simulink model "mfordmodel_v1"  (R2023a)
settings: Solver=ode45  StartTime=0.0  StopTime=10.0  RelTol=1e-3  EnableMultiTasking=on
undefined symbols (not defined in the file): ABV_RATIO_SW, AC_OFF_DLY, ACLOD, AUTO_TRNS_SW, BRAKE_DNDT_X, BZZRPM, BZZRPM_ALT, BZZTM, BZZTM_ALT, CMD_LITOFF, CMD_STABLE, CO_ST_ECT__A, COOL_BASE, DAS_BKDLY_A, DAS_CNT, DAS_CTDLY, DAS_LC_SW__A, DASCLP_5INH, DASCTL, DASMHYST, DASMPH, DEBYCP, DES_BASE, DPNEU_MUL, DSDRPM_DN_TC, DSDRPM_OFF, DSDRPM_UP_TC, EDF_DELAY, EDFHP, ETC_CL_TP, ETC_HP, GR_CM_CREEP, HCAM_ACT_CLP, HEDFHP, HEDFRPM, HICAM_PS, IAC_CAL_SW, IAC_ER_TM1, IAC_ER_TM2, IAC_ER_TM4, IAC_HI_LIM__A, IAC_ISFL_OBD, IAC_KAM_SW, IAC_LO_LIM__A, IAC_MON_TM, IAC_OT_REQ, IAC_RUN_TM, IAC_TP_OBD, IAC_TR_DAS, IAC_TST_DC, ID_DAS__A, ID_NOVS__A, IDVS_CH__A, IDVS_SL__A, IPSI_SW, IPSIDLY, IS_DRBASE__A, IS_DRBASE_A__A, IS_NUBASE__A, IS_NUBASE_A__A ... (+35)
libraries: simulink x2
(part 5 of 12)

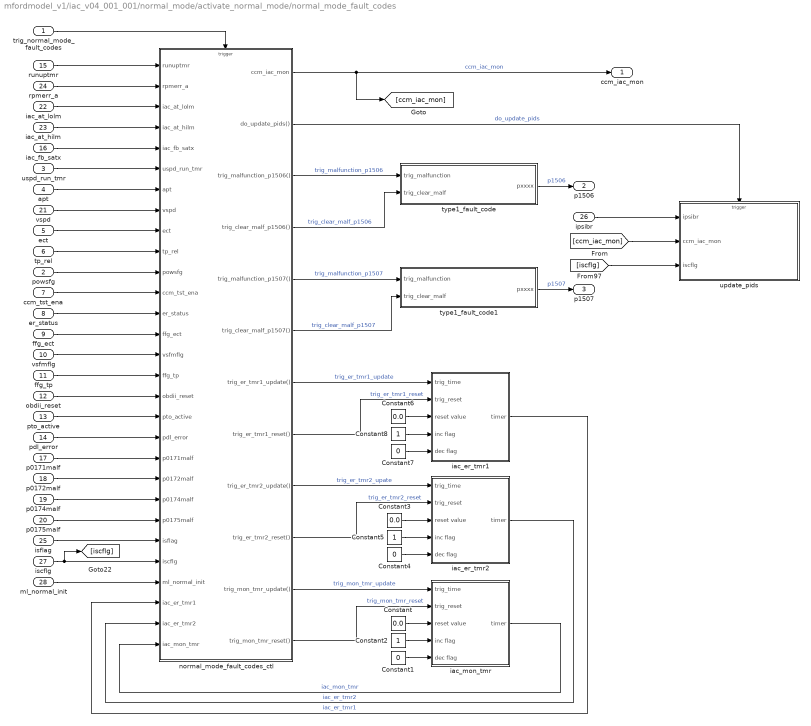
== system mfordmodel_v1/iac_v04_001_001/normal_mode/activate_normal_mode/normal_mode_fault_codes ==
  trig_normal_mode_fault_codes : Inport
  powsfg : Inport  Port=2
  uspd_run_tmr : Inport  Port=3
  apt : Inport  Port=4
  ect : Inport  Port=5
  tp_rel : Inport  Port=6
  ccm_tst_ena : Inport  Port=7
  er_status : Inport  Port=8
  ffg_ect : Inport  Port=9
  vsfmflg : Inport  Port=10
  ffg_tp : Inport  Port=11
  obdii_reset : Inport  Port=12
  pto_active : Inport  Port=13
  pdl_error : Inport  Port=14
  runuptmr : Inport  Port=15
  iac_fb_satx : Inport  Port=16
  p0171malf : Inport  Port=17
  p0172malf : Inport  Port=18
  p0174malf : Inport  Port=19
  p0175malf : Inport  Port=20
  vspd : Inport  Port=21
  iac_at_lolm : Inport  Port=22
  iac_at_hilm : Inport  Port=23
  rpmerr_a : Inport  Port=24
  isflag : Inport  Port=25
  ipsibr : Inport  Port=26
  iscflg : Inport  Port=27
  ml_normal_init : Inport  Port=28
  Constant : Constant  Value=0.0
  Constant1 : Constant  Value=0
  Constant2 : Constant
  Constant3 : Constant  Value=0.0
  Constant4 : Constant  Value=0
  Constant5 : Constant
  Constant6 : Constant  Value=0.0
  Constant7 : Constant  Value=0
  Constant8 : Constant
  iac_er_tmr1 : Subsystem  mask(TIMER){timer_name=iac_er_tmr1, init_value=0, clipped=off, tmin=, tmax=, unit_str=seconds}
      mask prompts: timer_name "Enter Timer Name"; init_value "initial TIMER value (in seconds)"; clipped "Clip timer?"; tmin "Minimum clip"; tmax "Maximum clip"; unit_str "Select timer units"
      mask help: Acts as a timer. Can count up, down, hold, or reset to zero. The required inputs are a timer function call, a reset function call, a reset value, an increment flag, and a decrement flag. Timer initial value, max and min clip values and timer name are selected below.
      mask init: same as mfordmodel_v1/iac_v04_001_001/normal_mode/activate_feedforward/ac_ppm_tmr
      mask Help:
      | <b><font size="+2">Input/Output Ports</font></b><br>
      | <p>
      | <b>Trig_timer:</b><br>
      | Connect a function call input to the 'trig_timer' port.  A function call passed through this port will activate the TIMER tool.  Activation updates the TIMER output.
      | <p>
      | <b>Trig_reset:</b><br>
      | Connect a function call input to the 'trig_reset' port.  A function call passed through this port will activate the TIMER tool.  Activation resets the TIMER output to the value passed to the 'reset_value' port.
      | <p>
      | <b>Reset_value:</b><br>
      | When 'trig_reset' is activated, the TIMER value will be reset to the real value passed to this input.
      | <p>
      | <b>Increment_flag and decrement_flag:</b><br>
      | If 'increment_flag' is 1 and 'decrement_flag' is 0, TIMER counts up.
      | If 'decrement_flag' is 1 and 'increment_flag' is 0, TIMER counts down.
      | If the flags are both 0 or both 1, TIMER holds its current value.
      | <p>
      | <b><font size="+2">Parameter Selection:</font></b>
      | <p>
      | <b>Initial TIMER Value:</b><br>
      | TIMER will begin at specified value.  Enter in seconds.
      mask TypeOptions unit_str: seconds | milliseconds
      mask Display:
      | plot( [0.3 0.45 0.55 0.7], [0.4 0.4 0.6 0.6])
      | plot( [ .475 .435 .415  .4 .4  .415 .435 .475  .525 .565 .585 .6 .6  ...
      | .585 .565 .525 .475], [.9  .885 .865  .825 .775 .735 .715  .7 .7 ...
      | .715 .735 .775 .825  .865 .885 .9 .9] )
      | plot( [.5 .5], [.89 .87])
      | plot( [.5 .5], [.71 .73])
      | plot( [.41 .43], [.8 .8])
      | plot( [.57 .59], [.8 .8])
      | plot( [.5 .5], [.8 .89])
      | plot( [.49 .5 .51], [.88 .89 .88] )
      | plot( [.5 .555], [.8 .825] )
      | plot( [.535 .555 .555], [.825 .825 .815])
      | text(0.35, 0.35, min_text)
      | text(0.6, 0.7,max_text)
      | text( 0.35, .95, timer_name)
  iac_er_tmr2 : Subsystem  mask(TIMER){timer_name=iac_er_tmr2, init_value=0, clipped=off, tmin=, tmax=, unit_str=seconds}
      mask prompts: timer_name "Enter Timer Name"; init_value "initial TIMER value (in seconds)"; clipped "Clip timer?"; tmin "Minimum clip"; tmax "Maximum clip"; unit_str "Select timer units"
      mask help: Acts as a timer. Can count up, down, hold, or reset to zero. The required inputs are a timer function call, a reset function call, a reset value, an increment flag, and a decrement flag. Timer initial value, max and min clip values and timer name are selected below.
      mask init: same as mfordmodel_v1/iac_v04_001_001/normal_mode/activate_feedforward/ac_ppm_tmr
      mask Help:
      | <b><font size="+2">Input/Output Ports</font></b><br>
      | <p>
      | <b>Trig_timer:</b><br>
      | Connect a function call input to the 'trig_timer' port.  A function call passed through this port will activate the TIMER tool.  Activation updates the TIMER output.
      | <p>
      | <b>Trig_reset:</b><br>
      | Connect a function call input to the 'trig_reset' port.  A function call passed through this port will activate the TIMER tool.  Activation resets the TIMER output to the value passed to the 'reset_value' port.
      | <p>
      | <b>Reset_value:</b><br>
      | When 'trig_reset' is activated, the TIMER value will be reset to the real value passed to this input.
      | <p>
      | <b>Increment_flag and decrement_flag:</b><br>
      | If 'increment_flag' is 1 and 'decrement_flag' is 0, TIMER counts up.
      | If 'decrement_flag' is 1 and 'increment_flag' is 0, TIMER counts down.
      | If the flags are both 0 or both 1, TIMER holds its current value.
      | <p>
      | <b><font size="+2">Parameter Selection:</font></b>
      | <p>
      | <b>Initial TIMER Value:</b><br>
      | TIMER will begin at specified value.  Enter in seconds.
      mask TypeOptions unit_str: seconds | milliseconds
      mask Display:
      | plot( [0.3 0.45 0.55 0.7], [0.4 0.4 0.6 0.6])
      | plot( [ .475 .435 .415  .4 .4  .415 .435 .475  .525 .565 .585 .6 .6  ...
      | .585 .565 .525 .475], [.9  .885 .865  .825 .775 .735 .715  .7 .7 ...
      | .715 .735 .775 .825  .865 .885 .9 .9] )
      | plot( [.5 .5], [.89 .87])
      | plot( [.5 .5], [.71 .73])
      | plot( [.41 .43], [.8 .8])
      | plot( [.57 .59], [.8 .8])
      | plot( [.5 .5], [.8 .89])
      | plot( [.49 .5 .51], [.88 .89 .88] )
      | plot( [.5 .555], [.8 .825] )
      | plot( [.535 .555 .555], [.825 .825 .815])
      | text(0.35, 0.35, min_text)
      | text(0.6, 0.7,max_text)
      | text( 0.35, .95, timer_name)
  iac_mon_tmr : Subsystem  mask(TIMER){timer_name=iac_mon_tmr, init_value=0, clipped=off, tmin=, tmax=, unit_str=seconds}
      mask prompts: timer_name "Enter Timer Name"; init_value "initial TIMER value (in seconds)"; clipped "Clip timer?"; tmin "Minimum clip"; tmax "Maximum clip"; unit_str "Select timer units"
      mask help: Acts as a timer. Can count up, down, hold, or reset to zero. The required inputs are a timer function call, a reset function call, a reset value, an increment flag, and a decrement flag. Timer initial value, max and min clip values and timer name are selected below.
      mask init: same as mfordmodel_v1/iac_v04_001_001/normal_mode/activate_feedforward/ac_ppm_tmr
      mask Help:
      | <b><font size="+2">Input/Output Ports</font></b><br>
      | <p>
      | <b>Trig_timer:</b><br>
      | Connect a function call input to the 'trig_timer' port.  A function call passed through this port will activate the TIMER tool.  Activation updates the TIMER output.
      | <p>
      | <b>Trig_reset:</b><br>
      | Connect a function call input to the 'trig_reset' port.  A function call passed through this port will activate the TIMER tool.  Activation resets the TIMER output to the value passed to the 'reset_value' port.
      | <p>
      | <b>Reset_value:</b><br>
      | When 'trig_reset' is activated, the TIMER value will be reset to the real value passed to this input.
      | <p>
      | <b>Increment_flag and decrement_flag:</b><br>
      | If 'increment_flag' is 1 and 'decrement_flag' is 0, TIMER counts up.
      | If 'decrement_flag' is 1 and 'increment_flag' is 0, TIMER counts down.
      | If the flags are both 0 or both 1, TIMER holds its current value.
      | <p>
      | <b><font size="+2">Parameter Selection:</font></b>
      | <p>
      | <b>Initial TIMER Value:</b><br>
      | TIMER will begin at specified value.  Enter in seconds.
      mask TypeOptions unit_str: seconds | milliseconds
      mask Display:
      | plot( [0.3 0.45 0.55 0.7], [0.4 0.4 0.6 0.6])
      | plot( [ .475 .435 .415  .4 .4  .415 .435 .475  .525 .565 .585 .6 .6  ...
      | .585 .565 .525 .475], [.9  .885 .865  .825 .775 .735 .715  .7 .7 ...
      | .715 .735 .775 .825  .865 .885 .9 .9] )
      | plot( [.5 .5], [.89 .87])
      | plot( [.5 .5], [.71 .73])
      | plot( [.41 .43], [.8 .8])
      | plot( [.57 .59], [.8 .8])
      | plot( [.5 .5], [.8 .89])
      | plot( [.49 .5 .51], [.88 .89 .88] )
      | plot( [.5 .555], [.8 .825] )
      | plot( [.535 .555 .555], [.825 .825 .815])
      | text(0.35, 0.35, min_text)
      | text(0.6, 0.7,max_text)
      | text( 0.35, .95, timer_name)
  normal_mode_fault_codes_ctl : Stateflow chart  TreatAsAtomicUnit=on
  type1_fault_code : Subsystem  mask(fault code){pcode=1506, ms=CCM}
      mask prompts: pcode "Code Number (e.g. 1234)"; ms "System ID"
      mask help: Gereric Fault Code - NOT functional
      mask init:
      | if (pcode == 'xxxx')
      | pcode_num = 0;
      | else
      | pcode_num = str2num(pcode);
      | end
      | mon_select=eval('ms');
      mask TypeOptions ms: CCM | CAT | PURG | SAIR | EGR | EGO | COOL | FCAP | P0456
      mask Display: fprintf('P%s\n%s',pcode,ms);
  type1_fault_code1 : Subsystem  mask(fault code){pcode=1507, ms=CCM}
      mask prompts: pcode "Code Number (e.g. 1234)"; ms "System ID"
      mask help: Gereric Fault Code - NOT functional
      mask init:
      | if (pcode == 'xxxx')
      | pcode_num = 0;
      | else
      | pcode_num = str2num(pcode);
      | end
      | mon_select=eval('ms');
      mask TypeOptions ms: CCM | CAT | PURG | SAIR | EGR | EGO | COOL | FCAP | P0456
      mask Display: fprintf('P%s\n%s',pcode,ms);
  update_pids : Subsystem  TreatAsAtomicUnit=on  mask(update_pids){}
      mask help: Update the specified PIDS.
      mask Display:
      | disp('
      | J2190_0x095D = ccm_iac_mon\n
      | J2190_0x097A = ipsibr               \n
      | J2190_0x097B = iscflg                \n')
  ccm_iac_mon : Outport
  p1506 : Outport  Port=2
  p1507 : Outport  Port=3
  wires:
  trig_normal_mode_fault_codes/1 -> normal_mode_fault_codes_ctl/Trigger
  normal_mode_fault_codes_ctl/7(trig_er_tmr1_update()) -> iac_er_tmr1/1(trig_time)  "trig_er_tmr1_update"
  normal_mode_fault_codes_ctl/8(trig_er_tmr1_reset()) -> iac_er_tmr1/2(trig_reset)  "trig_er_tmr1_reset"
  normal_mode_fault_codes_ctl/3(trig_malfunction_p1506()) -> type1_fault_code/1(trig_malfunction)  "trig_malfunction_p1506"
  normal_mode_fault_codes_ctl/4(trig_clear_malf_p1506()) -> type1_fault_code/2(trig_clear_malf)  "trig_clear_malf_p1506"
  normal_mode_fault_codes_ctl/5(trig_malfunction_p1507()) -> type1_fault_code1/1(trig_malfunction)  "trig_malfunction_p1507"
  normal_mode_fault_codes_ctl/6(trig_clear_malf_p1507()) -> type1_fault_code1/2(trig_clear_malf)  "trig_clear_malf_p1507"
  normal_mode_fault_codes_ctl/11(trig_mon_tmr_update()) -> iac_mon_tmr/1(trig_time)  "trig_mon_tmr_update"
  normal_mode_fault_codes_ctl/12(trig_mon_tmr_reset()) -> iac_mon_tmr/2(trig_reset)  "trig_mon_tmr_reset"
  normal_mode_fault_codes_ctl/10(trig_er_tmr2_reset()) -> iac_er_tmr2/2(trig_reset)  "trig_er_tmr2_reset"
  normal_mode_fault_codes_ctl/9(trig_er_tmr2_update()) -> iac_er_tmr2/1(trig_time)  "trig_er_tmr2_upate"
  iac_mon_tmr/1(timer) -> normal_mode_fault_codes_ctl/29(iac_mon_tmr)  "iac_mon_tmr"
  iac_er_tmr2/1(timer) -> normal_mode_fault_codes_ctl/28(iac_er_tmr2)  "iac_er_tmr2"
  iac_er_tmr1/1(timer) -> normal_mode_fault_codes_ctl/27(iac_er_tmr1)  "iac_er_tmr1"
  normal_mode_fault_codes_ctl/1(ccm_iac_mon) -> ccm_iac_mon/1, [ccm_iac_mon]  "ccm_iac_mon"
  Constant/1 -> iac_mon_tmr/3(reset value)
  Constant1/1 -> iac_mon_tmr/5(dec flag)
  Constant2/1 -> iac_mon_tmr/4(inc flag)
  Constant4/1 -> iac_er_tmr2/5(dec flag)
  Constant3/1 -> iac_er_tmr2/3(reset value)
  Constant5/1 -> iac_er_tmr2/4(inc flag)
  Constant6/1 -> iac_er_tmr1/3(reset value)
  Constant7/1 -> iac_er_tmr1/5(dec flag)
  Constant8/1 -> iac_er_tmr1/4(inc flag)
  normal_mode_fault_codes_ctl/2(do_update_pids()) -> update_pids/Trigger  "do_update_pids"
  iscflg/1 -> [iscflg], normal_mode_fault_codes_ctl/25(iscflg)
  ml_normal_init/1 -> normal_mode_fault_codes_ctl/26(ml_normal_init)
  runuptmr/1 -> normal_mode_fault_codes_ctl/1(runuptmr)
  rpmerr_a/1 -> normal_mode_fault_codes_ctl/2(rpmerr_a)
  iac_fb_satx/1 -> normal_mode_fault_codes_ctl/5(iac_fb_satx)
  iac_at_lolm/1 -> normal_mode_fault_codes_ctl/3(iac_at_lolm)
  iac_at_hilm/1 -> normal_mode_fault_codes_ctl/4(iac_at_hilm)
  isflag/1 -> normal_mode_fault_codes_ctl/24(isflag)
  powsfg/1 -> normal_mode_fault_codes_ctl/11(powsfg)
  uspd_run_tmr/1 -> normal_mode_fault_codes_ctl/6(uspd_run_tmr)
  apt/1 -> normal_mode_fault_codes_ctl/7(apt)
  vspd/1 -> normal_mode_fault_codes_ctl/8(vspd)
  ect/1 -> normal_mode_fault_codes_ctl/9(ect)
  tp_rel/1 -> normal_mode_fault_codes_ctl/10(tp_rel)
  ccm_tst_ena/1 -> normal_mode_fault_codes_ctl/12(ccm_tst_ena)
  er_status/1 -> normal_mode_fault_codes_ctl/13(er_status)
  ffg_ect/1 -> normal_mode_fault_codes_ctl/14(ffg_ect)
  vsfmflg/1 -> normal_mode_fault_codes_ctl/15(vsfmflg)
  ffg_tp/1 -> normal_mode_fault_codes_ctl/16(ffg_tp)
  obdii_reset/1 -> normal_mode_fault_codes_ctl/17(obdii_reset)
  pto_active/1 -> normal_mode_fault_codes_ctl/18(pto_active)
  pdl_error/1 -> normal_mode_fault_codes_ctl/19(pdl_error)
  p0171malf/1 -> normal_mode_fault_codes_ctl/20(p0171malf)
  p0172malf/1 -> normal_mode_fault_codes_ctl/21(p0172malf)
  p0174malf/1 -> normal_mode_fault_codes_ctl/22(p0174malf)
  p0175malf/1 -> normal_mode_fault_codes_ctl/23(p0175malf)
  type1_fault_code/1(pxxxx) -> p1506/1  "p1506"
  type1_fault_code1/1(pxxxx) -> p1507/1  "p1507"
  [iscflg] -> update_pids/3(iscflg)
  ipsibr/1 -> update_pids/1(ipsibr)
  [ccm_iac_mon] -> update_pids/2(ccm_iac_mon)

== system mfordmodel_v1/iac_v04_001_001/normal_mode/activate_normal_mode/output_flow_calc ==
  note: Note: Enable 'C-Like' bit
      | operations when Unit testing.
  note: UNIT TESTING NOTE: This module calculates "abv_flowrate"
      | and expects to see the modified value in the decision logic
      | "output_flow_calc_ctl" for determining the correct level of
      |  "iac_at_lolm & iac_at_hilm". Since "abv_flowrate" is a
      | merged parameter the model correctly has the merged
      | value "abv_flowrate_in" connected as an input to the decision
      | logic. However, since MatLab does not allow an input of a
      | merge block to be connected to more than one element,
      | it must  be manually wired to the state chart input for portions
      |  of the model unit test that utilize the limit logic.
      | ie, (P1506 & P1507 control).
  trig_output_flow_calc : Inport
  abv_percent : Inport  Port=2
  tr_res : Inport  Port=3
  tr_abs : Inport  Port=4
  pg_air : Inport  Port=5
  load : Inport  Port=6
  bp : Inport  Port=7
  engine_speed : Inport  Port=8
  act : Inport  Port=9
  map : Inport  Port=10
  abv_status : Inport  Port=11
  desmaf_pre : Inport  Port=12
  idle_ppm : Inport  Port=13
  isckam : Inport  Port=14
  ipsibr : Inport  Port=15
  isflag : Inport  Port=16
  abv_flowrate_in : Inport  Port=17
  abv_ratio_in : Inport  Port=18
  iac_inf_amb : Inport  Port=19
  desmaf_calc : Subsystem  TreatAsAtomicUnit=on
  output_flow_calc_ctl : Stateflow chart  TreatAsAtomicUnit=on
  tr_dsdrpm_calc : Subsystem  Description=test  TreatAsAtomicUnit=on  mask(tr_dsdrpm_calc){}
      mask help: TBD
      mask Display:
      | fprintf('ml_tr_dsdrpm_calc =
      | tr_abs - tr_res')
  abv_ratio : Outport
  abv_flowrate : Outport  Port=2
  iac_at_lolm : Outport  Port=3
  iac_at_hilm : Outport  Port=4
  iac_op_frac : Outport  Port=5
  wires:
  trig_output_flow_calc/1 -> output_flow_calc_ctl/Trigger
  output_flow_calc_ctl/2(iac_at_hilm) -> iac_at_hilm/1  "iac_at_hilm"
  output_flow_calc_ctl/1(iac_at_lolm) -> iac_at_lolm/1  "iac_at_lolm"
  abv_status/1 -> output_flow_calc_ctl/1(abv_status)
  output_flow_calc_ctl/9(do_tr_dsdrpm_calc()) -> tr_dsdrpm_calc/Trigger  "do_tr_dsdrpm_calc"
  tr_res/1 -> tr_dsdrpm_calc/2(tr_res)
  tr_abs/1 -> tr_dsdrpm_calc/1(tr_abs)
  tr_dsdrpm_calc/1(ml_tr_dsdrpm_calc) -> output_flow_calc_ctl/4(ml_tr_dsdrpm_calc), desmaf_calc/6(ml_tr_dsdrpm_calc)
  [do_desmaf_calc] -> desmaf_calc/Trigger
  output_flow_calc_ctl/3(ml_tr_dsdrpm_sw) -> desmaf_calc/1(ml_tr_dsdrpm_sw)  "ml_tr_dsdrpm_sw"
  output_flow_calc_ctl/5(ml_tr_das_sw) -> desmaf_calc/3(ml_tr_das_sw)  "ml_tr_das_sw"
  output_flow_calc_ctl/6(ml_ratio_sw) -> desmaf_calc/4(ml_ratio_sw)  "ml_ratio_sw"
  output_flow_calc_ctl/4(ml_flowrate_sw) -> desmaf_calc/2(ml_flowrate_sw)  "ml_flowrate_sw"
  output_flow_calc_ctl/8(do_desmaf_calc()) -> [do_desmaf_calc]  "do_desmaf_calc"
  isflag/1 -> output_flow_calc_ctl/2(isflag)
  output_flow_calc_ctl/7(ml_isflag_sw) -> desmaf_calc/5(ml_isflag_sw)  "ml_isflag_sw"
  abv_flowrate_in/1 -> output_flow_calc_ctl/3(abv_flowrate)
  desmaf_pre/1 -> desmaf_calc/7(desmaf_pre)
  ipsibr/1 -> desmaf_calc/9(ipsibr)
  idle_ppm/1 -> desmaf_calc/8(idle_ppm)
  isckam/1 -> desmaf_calc/10(isckam)
  map/1 -> desmaf_calc/11(map)
  bp/1 -> desmaf_calc/12(bp)
  engine_speed/1 -> desmaf_calc/15(engine_speed)
  load/1 -> desmaf_calc/16(load)
  act/1 -> desmaf_calc/14(act)
  pg_air/1 -> desmaf_calc/13(pg_air)
  abv_percent/1 -> desmaf_calc/17(abv_percent)
  abv_ratio_in/1 -> desmaf_calc/18(abv_ratio_in)
  desmaf_calc/1(iac_op_frac) -> iac_op_frac/1
  desmaf_calc/2(abv_ratio) -> abv_ratio/1
  desmaf_calc/3(abv_flowrate) -> abv_flowrate/1
  iac_inf_amb/1 -> desmaf_calc/19(iac_inf_amb)

== system mfordmodel_v1/iac_v04_001_001/normal_mode/iscflg_module/das_min_clip ==
  trig_das_min_clip_daspot : Inport
  trig_das_min_clip_prepos : Inport  Port=2
  dndsup : Inport  Port=3
  ndsflg : Inport  Port=4
  flg_crv_lk : Inport  Port=5
  dsdrpm : Inport  Port=6
  engine_speed : Inport  Port=7
  ptctfg : Inport  Port=8
  tfmflg : Inport  Port=9
  apt : Inport  Port=10
  flg_dasmnq : Inport  Port=11
  gear5tmr : Inport  Port=12
  das_ctr : Inport  Port=13
  dndt_das : Inport  Port=14
  iac_dlt_time : Inport  Port=15
  idle_ppm_in : Inport  Port=16
  gear5th : Inport  Port=17
  Gain : Gain  SaturateOnIntegerOverflow=on  OutDataTypeStr=Inherit: Same as input  ParamDataTypeStr=Inherit: Same as input
  Gain1 : Gain  SaturateOnIntegerOverflow=on  OutDataTypeStr=Inherit: Same as input  ParamDataTypeStr=Inherit: Same as input
  MinMax : MinMax  Function=max  Inputs=2  InputSameDT=on  SaturateOnIntegerOverflow=on
  Mux : Mux  Inputs=2
  das_min_clip_ctl : Stateflow chart  TreatAsAtomicUnit=on
  functions : Subsystem  TreatAsAtomicUnit=on
  daspot : Outport
  das_min_clp : Outport  Port=2
  idle_ppm : Outport  Port=3
  n_ratch : Outport  Port=4
  wires:
  das_min_clip_ctl/3(n_ratch) -> n_ratch/1, functions/1(n_ratch)  "n_ratch"
  MinMax/1 -> Gain1/1, Gain/1  "idle_ppm"
  Gain1/1 -> idle_ppm/1  "idle_ppm"
  Gain/1 -> daspot/1  "daspot"
  [idle_ppm_in] -> MinMax/2
  das_min_clip_ctl/1(das_min_clp) -> das_min_clp/1, MinMax/1  "das_min_clp"
  gear5th/1 -> das_min_clip_ctl/13(gear5th)
  idle_ppm_in/1 -> [idle_ppm_in], das_min_clip_ctl/12(idle_ppm_in)
  flg_crv_lk/1 -> das_min_clip_ctl/7(flg_crv_lk)
  tfmflg/1 -> das_min_clip_ctl/5(tfmflg)
  ptctfg/1 -> das_min_clip_ctl/3(ptctfg)
  dndsup/1 -> das_min_clip_ctl/1(dndsup)
  dndt_das/1 -> das_min_clip_ctl/11(dndt_das)
  das_ctr/1 -> das_min_clip_ctl/10(das_ctr)
  gear5tmr/1 -> das_min_clip_ctl/9(gear5tmr)
  flg_dasmnq/1 -> das_min_clip_ctl/8(flg_dasmnq)
  apt/1 -> das_min_clip_ctl/6(apt)
  ndsflg/1 -> das_min_clip_ctl/4(ndsflg)
  engine_speed/1 -> das_min_clip_ctl/2(engine_speed)
  iac_dlt_time/1 -> functions/3(iac_dlt_time)
  das_min_clip_ctl/2(dasl_min_clp) -> functions/2(dasl_min_clp)  "dasl_min_clp"
  functions/2(ml_rolav_llc) -> das_min_clip_ctl/21(ml_rolav_llc)
  functions/3(ml_rolav_l) -> das_min_clip_ctl/20(ml_rolav_l)
  functions/4(ml_rolav_h) -> das_min_clip_ctl/19(ml_rolav_h)
  functions/9(ml_fn894hlc) -> das_min_clip_ctl/14(ml_fn894hlc)
  functions/8(ml_fn894llc) -> das_min_clip_ctl/15(ml_fn894llc)
  functions/7(ml_fn894h) -> das_min_clip_ctl/16(ml_fn894h)
  functions/6(ml_fn894l) -> das_min_clip_ctl/17(ml_fn894l)
  functions/5(ml_fn894) -> das_min_clip_ctl/18(ml_fn894)
  dsdrpm/1 -> functions/4(dsdrpm)
  functions/1(ml_rolav_hlc) -> das_min_clip_ctl/22(ml_rolav_hlc)
  trig_das_min_clip_prepos/1 -> Mux/2
  trig_das_min_clip_daspot/1 -> Mux/1
  Mux/1 -> das_min_clip_ctl/Trigger
  das_min_clip_ctl/4(do_functions()) -> functions/Trigger  "do_functions"

== system mfordmodel_v1/iac_v04_001_001/normal_mode/iscflg_module/dashpot ==
  trig_activate_daspot_mode : Inport
  engine_speed : Inport  Port=2
  cttmr : Inport  Port=3
  apt : Inport  Port=4
  ndsflg : Inport  Port=5
  gr_cm : Inport  Port=6
  gr_old : Inport  Port=7
  pdl : Inport  Port=8
  vsbart : Inport  Port=9
  gr_cm_lst : Inport  Port=10
  igr_ds : Inport  Port=11
  flg_crv_lk : Inport  Port=12
  flg_sft_in : Inport  Port=13
  iac_dlt_time : Inport  Port=14
  idle_ppm_in : Inport  Port=15
  gear5th : Inport  Port=16
  dndt_das : Inport  Port=17
  ptctfg : Inport  Port=18
  Constant6 : Constant  Value=0
  Constant7 : Constant
  TIMER : Subsystem  mask(TIMER){timer_name=das_delay__A, init_value=0, clipped=on, tmin=0, tmax=inf, unit_str=seconds}
      mask prompts: timer_name "Enter Timer Name"; init_value "initial TIMER value (in seconds)"; clipped "Clip timer?"; tmin "Minimum clip"; tmax "Maximum clip"; unit_str "Select timer units"
      mask help: Acts as a timer. Can count up, down, hold, or reset to zero. The required inputs are a timer function call, a reset function call, a reset value, an increment flag, and a decrement flag. Timer initial value, max and min clip values and timer name are selected below.
      mask init: same as mfordmodel_v1/iac_v04_001_001/normal_mode/activate_feedforward/ac_ppm_tmr
      mask Help:
      | <b><font size="+2">Input/Output Ports</font></b><br>
      | <p>
      | <b>Trig_timer:</b><br>
      | Connect a function call input to the 'trig_timer' port.  A function call passed through this port will activate the TIMER tool.  Activation updates the TIMER output.
      | <p>
      | <b>Trig_reset:</b><br>
      | Connect a function call input to the 'trig_reset' port.  A function call passed through this port will activate the TIMER tool.  Activation resets the TIMER output to the value passed to the 'reset_value' port.
      | <p>
      | <b>Reset_value:</b><br>
      | When 'trig_reset' is activated, the TIMER value will be reset to the real value passed to this input.
      | <p>
      | <b>Increment_flag and decrement_flag:</b><br>
      | If 'increment_flag' is 1 and 'decrement_flag' is 0, TIMER counts up.
      | If 'decrement_flag' is 1 and 'increment_flag' is 0, TIMER counts down.
      | If the flags are both 0 or both 1, TIMER holds its current value.
      | <p>
      | <b><font size="+2">Parameter Selection:</font></b>
      | <p>
      | <b>Initial TIMER Value:</b><br>
      | TIMER will begin at specified value.  Enter in seconds.
      mask TypeOptions unit_str: seconds | milliseconds
      mask Display:
      | plot( [0.3 0.45 0.55 0.7], [0.4 0.4 0.6 0.6])
      | plot( [ .475 .435 .415  .4 .4  .415 .435 .475  .525 .565 .585 .6 .6  ...
      | .585 .565 .525 .475], [.9  .885 .865  .825 .775 .735 .715  .7 .7 ...
      | .715 .735 .775 .825  .865 .885 .9 .9] )
      | plot( [.5 .5], [.89 .87])
      | plot( [.5 .5], [.71 .73])
      | plot( [.41 .43], [.8 .8])
      | plot( [.57 .59], [.8 .8])
      | plot( [.5 .5], [.8 .89])
      | plot( [.49 .5 .51], [.88 .89 .88] )
      | plot( [.5 .555], [.8 .825] )
      | plot( [.535 .555 .555], [.825 .825 .815])
      | text(0.35, 0.35, min_text)
      | text(0.6, 0.7,max_text)
      | text( 0.35, .95, timer_name)
  activate_daspot_mode_ctl : Stateflow chart  TreatAsAtomicUnit=on
  daspot_calc : Subsystem  TreatAsAtomicUnit=on
  daspot_shift_trans_calc_ctl : Stateflow chart  TreatAsAtomicUnit=on
  function_calcs : Subsystem  TreatAsAtomicUnit=on
  trig_das_min_clip_daspot : Outport
  idle_ppm : Outport  Port=2
  das_ctr : Outport  Port=3
  wires:
  daspot_shift_trans_calc_ctl/2(das_tc__A) -> daspot_calc/5(das_tc__A)  "das_tc__A"
  daspot_shift_trans_calc_ctl/1(das_ppm__A) -> [das_ppm__A], daspot_calc/4(das_ppm__A)  "das_ppm__A"
  flg_crv_lk/1 -> activate_daspot_mode_ctl/8(flg_crv_lk)
  ptctfg/1 -> activate_daspot_mode_ctl/7(ptctfg)
  ndsflg/1 -> activate_daspot_mode_ctl/6(ndsflg)
  [engine_speed] -> activate_daspot_mode_ctl/9(engine_speed)
  [apt] -> activate_daspot_mode_ctl/10(apt)
  apt/1 -> [apt], daspot_shift_trans_calc_ctl/7(apt)
  [do_daspot_calc] -> daspot_calc/Trigger
  activate_daspot_mode_ctl/3(do_daspot_calc()) -> [do_daspot_calc]  "do_daspot_calc"
  [trig_dec_das_delay] -> TIMER/1(trig_time)
  activate_daspot_mode_ctl/5(trig_dec_das_delay()) -> [trig_dec_das_delay]  "trig_dec_das_delay"
  daspot_calc/1(idle_ppm) -> idle_ppm/1
  iac_dlt_time/1 -> daspot_calc/2(iac_dlt_time)
  idle_ppm_in/1 -> daspot_calc/3(idle_ppm_in)
  [trig_rst_das_delay] -> TIMER/2(trig_reset)
  Constant7/1 -> TIMER/5(dec flag)
  Constant6/1 -> TIMER/4(inc flag)
  daspot_shift_trans_calc_ctl/4(trig_rst_das_delay()) -> [trig_rst_das_delay]  "trig_rst_das_delay"
  [engine_speed] -> function_calcs/1(engine_speed)
  vsbart/1 -> [vsbart]
  engine_speed/1 -> [engine_speed]
  [vsbart] -> function_calcs/2(vsbart)
  daspot_shift_trans_calc_ctl/3(ml_das_delay) -> TIMER/3(reset value)  "ml_das_delay"
  TIMER/1(timer) -> [das_delay__A]  "das_delay__A"
  igr_ds/1 -> daspot_shift_trans_calc_ctl/1(igr_ds)
  pdl/1 -> daspot_shift_trans_calc_ctl/6(pdl)
  gr_cm/1 -> daspot_shift_trans_calc_ctl/4(gr_cm)
  flg_sft_in/1 -> daspot_shift_trans_calc_ctl/2(flg_sft_in)
  gr_cm_lst/1 -> daspot_shift_trans_calc_ctl/5(gr_cm_lst)
  gr_old/1 -> daspot_shift_trans_calc_ctl/3(gr_old)
  daspot_shift_trans_calc_ctl/5(do_function_calcs()) -> function_calcs/Trigger  "do_function_calcs"
  function_calcs/8(ml_fn899) -> daspot_shift_trans_calc_ctl/8(ml_fn899)
  function_calcs/7(ml_fnbo12) -> daspot_shift_trans_calc_ctl/9(ml_fnbo12)
  function_calcs/6(ml_fnbo13) -> daspot_shift_trans_calc_ctl/10(ml_fnbo13)
  function_calcs/5(ml_fnbo23) -> daspot_shift_trans_calc_ctl/11(ml_fnbo23)
  function_calcs/4(ml_fnbo24) -> daspot_shift_trans_calc_ctl/12(ml_fnbo24)
  function_calcs/3(ml_fnbo34) -> daspot_shift_trans_calc_ctl/13(ml_fnbo34)
  function_calcs/2(ml_fnbo35) -> daspot_shift_trans_calc_ctl/14(ml_fnbo35)
  function_calcs/1(ml_fnbo45) -> daspot_shift_trans_calc_ctl/15(ml_fnbo45)
  activate_daspot_mode_ctl/6(trig_daspot_shift_trans_calc()) -> daspot_shift_trans_calc_ctl/Trigger  "trig_daspot_shift_trans_calc"
  dndt_das/1 -> activate_daspot_mode_ctl/5(dndt_das)
  cttmr/1 -> activate_daspot_mode_ctl/4(cttmr)
  gear5th/1 -> activate_daspot_mode_ctl/3(gear5th)
  activate_daspot_mode_ctl/2(das_ctr) -> das_ctr/1  "das_ctr"
  activate_daspot_mode_ctl/4(trig_das_min_clip_daspot()) -> trig_das_min_clip_daspot/1  "trig_das_min_clip_daspot"
  activate_daspot_mode_ctl/1(ml_idle_ppm_sw) -> daspot_calc/1(ml_idle_ppm_sw)  "ml_idle_ppm_sw"
  trig_activate_daspot_mode/1 -> activate_daspot_mode_ctl/Trigger
  [das_delay__A] -> activate_daspot_mode_ctl/1(das_delay__A)
  [das_ppm__A] -> activate_daspot_mode_ctl/2(das_ppm__A)

== system mfordmodel_v1/iac_v04_001_001/normal_mode/iscflg_module/idle_drive_rpm_controller ==
  trig_idle_drive_rpm_controller : Inport
  ml_idrv_init_flg : Inport  Port=2
  iac_dlt_time : Inport  Port=3
  engine_speed : Inport  Port=4
  load : Inport  Port=5
  idle_drive_rpm_controller_ctl : Stateflow chart  TreatAsAtomicUnit=on
  idle_ppm_calc : Subsystem  TreatAsAtomicUnit=on
  idnerr_fil_calc : Subsystem  TreatAsAtomicUnit=on  mask(idnerr_fil_calc){}
      mask help: TBD
      mask Display:
      | disp('
      | ml_idnerr = (DSDRPM__A - engine_speed) \n\n
      | idnerr_fil = ROLAV (idnerr_fil, ml_idnerr,    \n
      | iac_dlt_time,  IDNERR_TC )       ')
  idle_ppm : Outport
  wires:
  idnerr_fil_calc/1(ml_idnerr) -> idle_ppm_calc/1(ml_idnerr)
  [do_idle_ppm_calc] -> idle_ppm_calc/Trigger
  idle_ppm_calc/1(idle_ppm) -> idle_ppm/1
  idle_ppm_calc/2(idnerr__A) -> [idnerr__A]
  [ml_init_sw] -> idle_ppm_calc/3(ml_init_sw)
  [ml_idnerr_sw] -> idle_ppm_calc/4(ml_idnerr_sw)
  load/1 -> idle_ppm_calc/5(load)
  idnerr_fil_calc/2(idnerr_fil) -> idle_drive_rpm_controller_ctl/2(idnerr_fil), idle_ppm_calc/2(idnerr_fil)
  iac_dlt_time/1 -> idnerr_fil_calc/3(iac_dlt_time)
  engine_speed/1 -> idnerr_fil_calc/2(engine_speed)
  [do_idnerr_fil_calc] -> idnerr_fil_calc/Trigger
  idle_drive_rpm_controller_ctl/1(ml_init_sw) -> idnerr_fil_calc/1(ml_init_sw), [ml_init_sw]  "ml_init_sw"
  idle_drive_rpm_controller_ctl/2(ml_idnerr_sw) -> [ml_idnerr_sw]  "ml_idnerr_sw"
  trig_idle_drive_rpm_controller/1 -> idle_drive_rpm_controller_ctl/Trigger
  ml_idrv_init_flg/1 -> idle_drive_rpm_controller_ctl/1(ml_idrv_init_flg)
  idle_drive_rpm_controller_ctl/3(do_idle_ppm_calc()) -> [do_idle_ppm_calc]  "do_idle_ppm_calc"
  idle_drive_rpm_controller_ctl/4(do_idnerr_fil_calc()) -> [do_idnerr_fil_calc]  "do_idnerr_fil_calc"
  [idnerr__A] -> idle_drive_rpm_controller_ctl/3(idnerr__A)

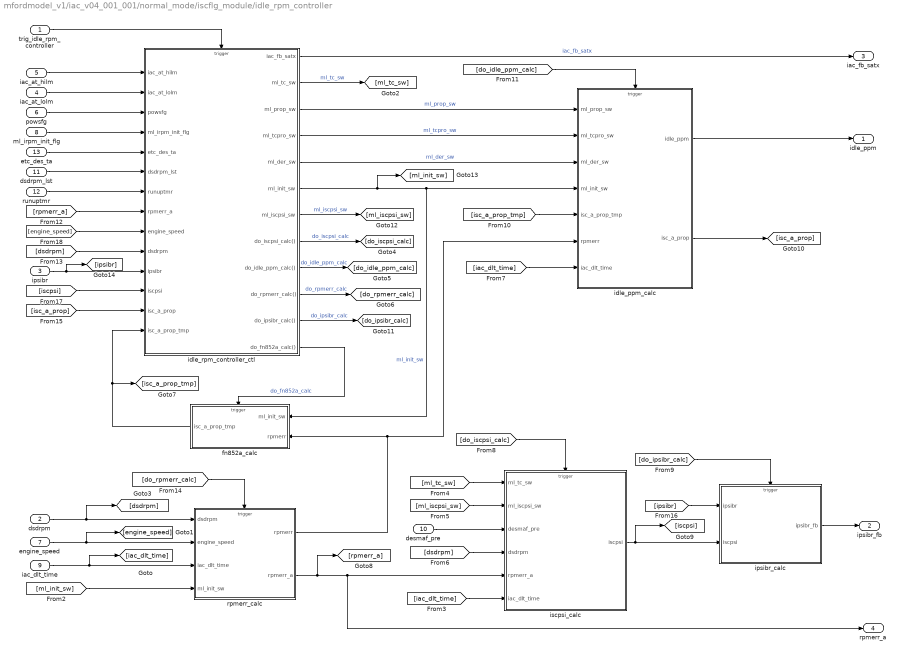
== system mfordmodel_v1/iac_v04_001_001/normal_mode/iscflg_module/idle_rpm_controller ==
  trig_idle_rpm_controller : Inport
  dsdrpm : Inport  Port=2
  ipsibr : Inport  Port=3
  iac_at_lolm : Inport  Port=4
  iac_at_hilm : Inport  Port=5
  powsfg : Inport  Port=6
  engine_speed : Inport  Port=7
  ml_irpm_init_flg : Inport  Port=8
  iac_dlt_time : Inport  Port=9
  desmaf_pre : Inport  Port=10
  dsdrpm_lst : Inport  Port=11
  runuptmr : Inport  Port=12
  etc_des_ta : Inport  Port=13
  fn852a_calc : Subsystem  TreatAsAtomicUnit=on
  idle_ppm_calc : Subsystem  TreatAsAtomicUnit=on
  idle_rpm_controller_ctl : Stateflow chart  TreatAsAtomicUnit=on
  ipsibr_calc : Subsystem  TreatAsAtomicUnit=on  mask(ipsibr_calc){}
      mask help: Calculate ipsibr feedback value.
      mask Display:
      | disp('
      | ipsibr_fb = ipsibr + iscpsi\n
      | ')
  iscpsi_calc : Subsystem  TreatAsAtomicUnit=on
  rpmerr_calc : Subsystem  TreatAsAtomicUnit=on
  idle_ppm : Outport
  ipsibr_fb : Outport  Port=2
  iac_fb_satx : Outport  Port=3
  rpmerr_a : Outport  Port=4
  wires:
  [engine_speed] -> idle_rpm_controller_ctl/9(engine_speed)
  engine_speed/1 -> [engine_speed], rpmerr_calc/2(engine_speed)
  powsfg/1 -> idle_rpm_controller_ctl/3(powsfg)
  iac_at_lolm/1 -> idle_rpm_controller_ctl/2(iac_at_lolm)
  iac_at_hilm/1 -> idle_rpm_controller_ctl/1(iac_at_hilm)
  ml_irpm_init_flg/1 -> idle_rpm_controller_ctl/4(ml_irpm_init_flg)
  etc_des_ta/1 -> idle_rpm_controller_ctl/5(etc_des_ta)
  dsdrpm_lst/1 -> idle_rpm_controller_ctl/6(dsdrpm_lst)
  idle_rpm_controller_ctl/7(ml_iscpsi_sw) -> [ml_iscpsi_sw]  "ml_iscpsi_sw"
  idle_rpm_controller_ctl/11(do_ipsibr_calc()) -> [do_ipsibr_calc]  "do_ipsibr_calc"
  idle_ppm_calc/2(isc_a_prop) -> [isc_a_prop]
  [do_idle_ppm_calc] -> idle_ppm_calc/Trigger
  [isc_a_prop_tmp] -> idle_ppm_calc/5(isc_a_prop_tmp)
  [iac_dlt_time] -> idle_ppm_calc/7(iac_dlt_time)
  idle_ppm_calc/1(idle_ppm) -> idle_ppm/1
  idle_rpm_controller_ctl/5(ml_der_sw) -> idle_ppm_calc/3(ml_der_sw)  "ml_der_sw"
  idle_rpm_controller_ctl/4(ml_tcpro_sw) -> idle_ppm_calc/2(ml_tcpro_sw)  "ml_tcpro_sw"
  idle_rpm_controller_ctl/3(ml_prop_sw) -> idle_ppm_calc/1(ml_prop_sw)  "ml_prop_sw"
  [iscpsi] -> idle_rpm_controller_ctl/12(iscpsi)
  trig_idle_rpm_controller/1 -> idle_rpm_controller_ctl/Trigger
  [do_ipsibr_calc] -> ipsibr_calc/Trigger
  ipsibr_calc/1(ipsibr_fb) -> ipsibr_fb/1
  runuptmr/1 -> idle_rpm_controller_ctl/7(runuptmr)
  [isc_a_prop] -> idle_rpm_controller_ctl/13(isc_a_prop)
  [do_rpmerr_calc] -> rpmerr_calc/Trigger
  iscpsi_calc/1(iscpsi) -> [iscpsi], ipsibr_calc/2(iscpsi)
  [dsdrpm] -> idle_rpm_controller_ctl/10(dsdrpm)
  desmaf_pre/1 -> iscpsi_calc/3(desmaf_pre)
  [rpmerr_a] -> idle_rpm_controller_ctl/8(rpmerr_a)
  rpmerr_calc/2(rpmerr_a) -> rpmerr_a/1, iscpsi_calc/5(rpmerr_a), [rpmerr_a]
  dsdrpm/1 -> [dsdrpm], rpmerr_calc/1(dsdrpm)
  [ml_init_sw] -> rpmerr_calc/4(ml_init_sw)
  iac_dlt_time/1 -> [iac_dlt_time], rpmerr_calc/3(iac_dlt_time)
  fn852a_calc/1(isc_a_prop_tmp) -> idle_rpm_controller_ctl/14(isc_a_prop_tmp), [isc_a_prop_tmp]
  idle_rpm_controller_ctl/10(do_rpmerr_calc()) -> [do_rpmerr_calc]  "do_rpmerr_calc"
  idle_rpm_controller_ctl/9(do_idle_ppm_calc()) -> [do_idle_ppm_calc]  "do_idle_ppm_calc"
  idle_rpm_controller_ctl/8(do_iscpsi_calc()) -> [do_iscpsi_calc]  "do_iscpsi_calc"
  [do_iscpsi_calc] -> iscpsi_calc/Trigger
  [dsdrpm] -> iscpsi_calc/4(dsdrpm)
  [ml_iscpsi_sw] -> iscpsi_calc/2(ml_iscpsi_sw)
  [ml_tc_sw] -> iscpsi_calc/1(ml_tc_sw)
  [iac_dlt_time] -> iscpsi_calc/6(iac_dlt_time)
  rpmerr_calc/1(rpmerr) -> idle_ppm_calc/6(rpmerr), fn852a_calc/2(rpmerr)
  idle_rpm_controller_ctl/1(iac_fb_satx) -> iac_fb_satx/1  "iac_fb_satx"
  idle_rpm_controller_ctl/2(ml_tc_sw) -> [ml_tc_sw]  "ml_tc_sw"
  idle_rpm_controller_ctl/12(do_fn852a_calc()) -> fn852a_calc/Trigger  "do_fn852a_calc"
  idle_rpm_controller_ctl/6(ml_init_sw) -> idle_ppm_calc/4(ml_init_sw), fn852a_calc/1(ml_init_sw), [ml_init_sw]  "ml_init_sw"
  ipsibr/1 -> idle_rpm_controller_ctl/11(ipsibr), [ipsibr]
  [ipsibr] -> ipsibr_calc/1(ipsibr)

== system mfordmodel_v1/iac_v04_001_001/normal_mode/iscflg_module/iscflg_modes ==
  note: Note: Make a direct connection
      | for "iscflg" from determine_iscflg_mode_ctl port 1
      | to activate_iscflg_mode_ctl input port 1 for unit
      | test purposes.
  trig_iscflg_modes : Inport
  engine_speed : Inport  Port=2
  vspd : Inport  Port=3
  novs_mtx__A : Inport  Port=4
  runuptmr : Inport  Port=5
  load : Inport  Port=6
  apt : Inport  Port=7
  accflg : Inport  Port=8
  dndsup : Inport  Port=9
  ndsflg : Inport  Port=10
  idle_ppm : Inport  Port=11
  ml_normal_init : Inport  Port=12
  iscflg_in : Inport  Port=13
  dsdrpm : Inport  Port=14
  1 : Subsystem  mask(TIMER){timer_name=isctmr, init_value=0, clipped=off, tmin=, tmax=, unit_str=seconds}
      mask prompts: timer_name "Enter Timer Name"; init_value "initial TIMER value (in seconds)"; clipped "Clip timer?"; tmin "Minimum clip"; tmax "Maximum clip"; unit_str "Select timer units"
      mask help: Acts as a timer. Can count up, down, hold, or reset to zero. The required inputs are a timer function call, a reset function call, a reset value, an increment flag, and a decrement flag. Timer initial value, max and min clip values and timer name are selected below.
      mask init: same as mfordmodel_v1/iac_v04_001_001/normal_mode/activate_feedforward/ac_ppm_tmr
      mask Help:
      | <b><font size="+2">Input/Output Ports</font></b><br>
      | <p>
      | <b>Trig_timer:</b><br>
      | Connect a function call input to the 'trig_timer' port.  A function call passed through this port will activate the TIMER tool.  Activation updates the TIMER output.
      | <p>
      | <b>Trig_reset:</b><br>
      | Connect a function call input to the 'trig_reset' port.  A function call passed through this port will activate the TIMER tool.  Activation resets the TIMER output to the value passed to the 'reset_value' port.
      | <p>
      | <b>Reset_value:</b><br>
      | When 'trig_reset' is activated, the TIMER value will be reset to the real value passed to this input.
      | <p>
      | <b>Increment_flag and decrement_flag:</b><br>
      | If 'increment_flag' is 1 and 'decrement_flag' is 0, TIMER counts up.
      | If 'decrement_flag' is 1 and 'increment_flag' is 0, TIMER counts down.
      | If the flags are both 0 or both 1, TIMER holds its current value.
      | <p>
      | <b><font size="+2">Parameter Selection:</font></b>
      | <p>
      | <b>Initial TIMER Value:</b><br>
      | TIMER will begin at specified value.  Enter in seconds.
      mask TypeOptions unit_str: seconds | milliseconds
      mask Display:
      | plot( [0.3 0.45 0.55 0.7], [0.4 0.4 0.6 0.6])
      | plot( [ .475 .435 .415  .4 .4  .415 .435 .475  .525 .565 .585 .6 .6  ...
      | .585 .565 .525 .475], [.9  .885 .865  .825 .775 .735 .715  .7 .7 ...
      | .715 .735 .775 .825  .865 .885 .9 .9] )
      | plot( [.5 .5], [.89 .87])
      | plot( [.5 .5], [.71 .73])
      | plot( [.41 .43], [.8 .8])
      | plot( [.57 .59], [.8 .8])
      | plot( [.5 .5], [.8 .89])
      | plot( [.49 .5 .51], [.88 .89 .88] )
      | plot( [.5 .555], [.8 .825] )
      | plot( [.535 .555 .555], [.825 .825 .815])
      | text(0.35, 0.35, min_text)
      | text(0.6, 0.7,max_text)
      | text( 0.35, .95, timer_name)
  2 : Subsystem  mask(TIMER){timer_name=settmr, init_value=0, clipped=off, tmin=, tmax=, unit_str=seconds}
      mask prompts: timer_name "Enter Timer Name"; init_value "initial TIMER value (in seconds)"; clipped "Clip timer?"; tmin "Minimum clip"; tmax "Maximum clip"; unit_str "Select timer units"
      mask help: Acts as a timer. Can count up, down, hold, or reset to zero. The required inputs are a timer function call, a reset function call, a reset value, an increment flag, and a decrement flag. Timer initial value, max and min clip values and timer name are selected below.
      mask init: same as mfordmodel_v1/iac_v04_001_001/normal_mode/activate_feedforward/ac_ppm_tmr
      mask Help:
      | <b><font size="+2">Input/Output Ports</font></b><br>
      | <p>
      | <b>Trig_timer:</b><br>
      | Connect a function call input to the 'trig_timer' port.  A function call passed through this port will activate the TIMER tool.  Activation updates the TIMER output.
      | <p>
      | <b>Trig_reset:</b><br>
      | Connect a function call input to the 'trig_reset' port.  A function call passed through this port will activate the TIMER tool.  Activation resets the TIMER output to the value passed to the 'reset_value' port.
      | <p>
      | <b>Reset_value:</b><br>
      | When 'trig_reset' is activated, the TIMER value will be reset to the real value passed to this input.
      | <p>
      | <b>Increment_flag and decrement_flag:</b><br>
      | If 'increment_flag' is 1 and 'decrement_flag' is 0, TIMER counts up.
      | If 'decrement_flag' is 1 and 'increment_flag' is 0, TIMER counts down.
      | If the flags are both 0 or both 1, TIMER holds its current value.
      | <p>
      | <b><font size="+2">Parameter Selection:</font></b>
      | <p>
      | <b>Initial TIMER Value:</b><br>
      | TIMER will begin at specified value.  Enter in seconds.
      mask TypeOptions unit_str: seconds | milliseconds
      mask Display:
      | plot( [0.3 0.45 0.55 0.7], [0.4 0.4 0.6 0.6])
      | plot( [ .475 .435 .415  .4 .4  .415 .435 .475  .525 .565 .585 .6 .6  ...
      | .585 .565 .525 .475], [.9  .885 .865  .825 .775 .735 .715  .7 .7 ...
      | .715 .735 .775 .825  .865 .885 .9 .9] )
      | plot( [.5 .5], [.89 .87])
      | plot( [.5 .5], [.71 .73])
      | plot( [.41 .43], [.8 .8])
      | plot( [.57 .59], [.8 .8])
      | plot( [.5 .5], [.8 .89])
      | plot( [.49 .5 .51], [.88 .89 .88] )
      | plot( [.5 .555], [.8 .825] )
      | plot( [.535 .555 .555], [.825 .825 .815])
      | text(0.35, 0.35, min_text)
      | text(0.6, 0.7,max_text)
      | text( 0.35, .95, timer_name)
  Constant3 : Constant  Value=0.0
  Constant4 : Constant  Value=0
  Constant5 : Constant
  Constant6 : Constant  Value=0.0
  Constant7 : Constant  Value=0
  Constant8 : Constant
  Mux : Mux  Inputs=2
  activate_iscflg_mode_ctl : Stateflow chart  TreatAsAtomicUnit=on
  determine_iscflg_mode_ctl : Stateflow chart  TreatAsAtomicUnit=on
  iscflg_modes_ctl : Stateflow chart  TreatAsAtomicUnit=on
  iscflg : Outport
  trig_activate_daspot_mode : Outport  Port=2
  trig_preposition : Outport  Port=3
  trig_idle_rpm_controller : Outport  Port=4
  trig_idle_drive_rpm_controller : Outport  Port=5
  ml_irpm_init_flg : Outport  Port=6
  ml_idrv_init_flg : Outport  Port=7
  daspot : Outport  Port=8
  id_mode : Outport  Port=9
  wires:
  activate_iscflg_mode_ctl/4(id_mode) -> id_mode/1  "id_mode"
  activate_iscflg_mode_ctl/3(daspot) -> daspot/1  "daspot"
  [iscflg] -> activate_iscflg_mode_ctl/1(iscflg)
  determine_iscflg_mode_ctl/1(iscflg) -> iscflg/1  "iscflg"
  iscflg_modes_ctl/3(trig_normal_reset()) -> Mux/2  "trig_normal_reset"
  iscflg_modes_ctl/2(trig_determine_iscflg_mode()) -> Mux/1  "trig_determine_iscflg_mode"
  Mux/1 -> determine_iscflg_mode_ctl/Trigger
  activate_iscflg_mode_ctl/2(ml_irpm_init_flg) -> ml_irpm_init_flg/1  "ml_irpm_init_flg"
  activate_iscflg_mode_ctl/1(ml_idrv_init_flg) -> ml_idrv_init_flg/1  "ml_idrv_init_flg"
  activate_iscflg_mode_ctl/8(trig_idle_drive_rpm_controller()) -> trig_idle_drive_rpm_controller/1  "trig_idle_drive_rpm_controller"
  activate_iscflg_mode_ctl/7(trig_idle_rpm_controller()) -> trig_idle_rpm_controller/1  "trig_idle_rpm_controller"
  activate_iscflg_mode_ctl/6(trig_preposition()) -> trig_preposition/1  "trig_preposition"
  activate_iscflg_mode_ctl/5(trig_activate_daspot_mode()) -> trig_activate_daspot_mode/1  "trig_activate_daspot_mode"
  ml_normal_init/1 -> iscflg_modes_ctl/1(ml_normal_init)
  iscflg_modes_ctl/1(trig_activate_iscflg_mode()) -> activate_iscflg_mode_ctl/Trigger  "trig_activate_iscflg_mode"
  trig_iscflg_modes/1 -> iscflg_modes_ctl/Trigger
  determine_iscflg_mode_ctl/2(trig_isctmr_reset()) -> 1/2(trig_reset)  "trig_isctmr_reset"
  determine_iscflg_mode_ctl/3(trig_isctmr_update()) -> 1/1(trig_time)  "trig_isctmr_update"
  Constant7/1 -> 1/5(dec flag)
  Constant8/1 -> 1/4(inc flag)
  Constant6/1 -> 1/3(reset value)
  1/1(timer) -> determine_iscflg_mode_ctl/13(isctmr)  "isctmr"
  determine_iscflg_mode_ctl/4(trig_settmr_reset()) -> 2/2(trig_reset)  "trig_settmr_reset"
  determine_iscflg_mode_ctl/5(trig_settmr_update()) -> 2/1(trig_time)  "trig_settmr_update"
  Constant4/1 -> 2/5(dec flag)
  Constant5/1 -> 2/4(inc flag)
  Constant3/1 -> 2/3(reset value)
  2/1(timer) -> determine_iscflg_mode_ctl/14(settmr)  "settmr"
  iscflg_in/1 -> [iscflg], determine_iscflg_mode_ctl/11(iscflg_in)
  novs_mtx__A/1 -> determine_iscflg_mode_ctl/10(novs_mtx__A)
  ndsflg/1 -> determine_iscflg_mode_ctl/9(ndsflg)
  accflg/1 -> determine_iscflg_mode_ctl/7(accflg)
  runuptmr/1 -> determine_iscflg_mode_ctl/6(runuptmr)
  idle_ppm/1 -> determine_iscflg_mode_ctl/8(idle_ppm)
  apt/1 -> determine_iscflg_mode_ctl/5(apt)
  dndsup/1 -> determine_iscflg_mode_ctl/4(dndsup)
  load/1 -> determine_iscflg_mode_ctl/3(load)
  vspd/1 -> determine_iscflg_mode_ctl/2(vspd)
  engine_speed/1 -> determine_iscflg_mode_ctl/1(engine_speed)
  dsdrpm/1 -> determine_iscflg_mode_ctl/12(dsdrpm)

== system mfordmodel_v1/iac_v04_001_001/normal_mode/iscflg_module/preposition ==
  trig_preposition : Inport
  dsdrpm : Inport  Port=2
  dndsup : Inport  Port=3
  engine_speed : Inport  Port=4
  ect : Inport  Port=5
  vspd : Inport  Port=6
  dstpbr : Inport  Port=7
  ratch : Inport  Port=8
  idle_ppm_calc : Subsystem  TreatAsAtomicUnit=on
  preposition_ctl : Stateflow chart  TreatAsAtomicUnit=on
  trig_das_min_clip_prepos : Outport
  idle_ppm : Outport  Port=2
  wires:
  preposition_ctl/2(trig_das_min_clip_prepos()) -> trig_das_min_clip_prepos/1  "trig_das_min_clip_prepos"
  [ml_mul_sw] -> idle_ppm_calc/1(ml_mul_sw)
  preposition_ctl/1(ml_mul_sw) -> [ml_mul_sw]  "ml_mul_sw"
  dndsup/1 -> preposition_ctl/1(dndsup)
  trig_preposition/1 -> preposition_ctl/Trigger
  preposition_ctl/3(do_idle_ppm_calc()) -> idle_ppm_calc/Trigger  "do_idle_ppm_calc"
  ratch/1 -> idle_ppm_calc/7(ratch)
  dstpbr/1 -> idle_ppm_calc/6(dstpbr)
  vspd/1 -> idle_ppm_calc/5(vspd)
  ect/1 -> idle_ppm_calc/4(ect)
  engine_speed/1 -> idle_ppm_calc/3(engine_speed)
  dsdrpm/1 -> idle_ppm_calc/2(dsdrpm)
  idle_ppm_calc/1(idle_ppm) -> idle_ppm/1

== system mfordmodel_v1/iac_v04_001_001/activate_desired_rpm/base_rpm_and_select_logic/dsdrpm_calc/ROLAV_TC_in_DT_in ==
  note: Using the first two terms of the series expansion:
      |
      |                     x                     x2
      |                                e   =  1  +  x  +  --  + ......
      |                                           2!
      |
      |       Simplifying, the exponential "f" becomes:
      |
      |                  - (FK_TMR/TC)              1
      |           f  =  1  -  e                    =  1  -  -------------  =  . . .
      |                                                    (FK_TMR/TC)
      |                           e
      |
      |                              1                      1
      |          f  =  1  -  ---------------------------------  =    ------------------- .
      |                                  1 + (FK_TMR / TC)       1 + (TC / FK_TMR)
  note: - (FK_TMR/TC)
      |                                    f  =  1  -  e
      |
      |       Where "f" is called the filter constant in the difference equation:
      |
      |                    new_average = f * new_value + (1 - f) * old_average
  note: new_average = [ (sample_interval)/(sample_interval + time_constant) ] * (new_value - old_ave) + old_ave
  new_value : Inport
  Tau : Inport  Port=2
  old_ave : Inport  Port=3
  delta_time : Inport  Port=4
  Elementary Math : Math  Operator=reciprocal  SignedPower=on
  Product : Product  Inputs=3  InputSameDT=on  RndMeth=Zero  SaturateOnIntegerOverflow=on  OutDataTypeStr=Inherit: Same as first input
  Sum : Sum  Inputs=-+  InputSameDT=on  SaturateOnIntegerOverflow=on  OutDataTypeStr=Inherit: Same as first input
  Sum1 : Sum  InputSameDT=on  SaturateOnIntegerOverflow=on  OutDataTypeStr=Inherit: Same as first input
  Sum2 : Sum  InputSameDT=on  SaturateOnIntegerOverflow=on  OutDataTypeStr=Inherit: Same as first input
  new_ave : Outport
  wires:
  delta_time/1 -> Product/2, Sum1/1
  Tau/1 -> Sum1/2
  Sum2/1 -> new_ave/1
  old_ave/1 -> Sum2/1, Sum/1
  Product/1 -> Sum2/2
  Sum/1 -> Product/1
  Elementary Math/1 -> Product/3
  Sum1/1 -> Elementary Math/1
  new_value/1 -> Sum/2

== system mfordmodel_v1/iac_v04_001_001/activate_desired_rpm/base_rpm_and_select_logic/dsdrpm_calc/pid ==
  data : Inport
  ctrl : Inport  Port=2
  Terminator : Terminator
  Terminator1 : Terminator
  wires:
  ctrl/1 -> Terminator1/1
  data/1 -> Terminator/1

== system mfordmodel_v1/iac_v04_001_001/activate_desired_rpm/base_rpm_and_select_logic/htr_core_rpm_calc/lookup_2d ==
  In1 : Inport
  Look-Up Table1 : Lookup  InputValues=calfunc.X  Table=calfunc.Y
  Saturation1 : Saturate  UpperLimit=max_x  LowerLimit=min_x
  Out1 : Outport
  wires:
  In1/1 -> Saturation1/1
  Saturation1/1 -> Look-Up Table1/1
  Look-Up Table1/1 -> Out1/1

== system mfordmodel_v1/iac_v04_001_001/activate_desired_rpm/base_rpm_and_select_logic/htr_core_rpm_calc/lookup_2d1 ==
  In1 : Inport
  Look-Up Table1 : Lookup  InputValues=calfunc.X  Table=calfunc.Y
  Saturation1 : Saturate  UpperLimit=max_x  LowerLimit=min_x
  Out1 : Outport
  wires:
  In1/1 -> Saturation1/1
  Saturation1/1 -> Look-Up Table1/1
  Look-Up Table1/1 -> Out1/1

== system mfordmodel_v1/iac_v04_001_001/activate_desired_rpm/hicam_rpm_request/fox_calcs/CONSTANT ==
  Constant : Constant  Value=const
  Out : Outport
  wires:
  Constant/1 -> Out/1

== system mfordmodel_v1/iac_v04_001_001/activate_desired_rpm/hicam_rpm_request/fox_calcs/lookup_2d ==
  In1 : Inport
  Look-Up Table1 : Lookup  InputValues=calfunc.X  Table=calfunc.Y
  Saturation1 : Saturate  UpperLimit=max_x  LowerLimit=min_x
  Out1 : Outport
  wires:
  In1/1 -> Saturation1/1
  Saturation1/1 -> Look-Up Table1/1
  Look-Up Table1/1 -> Out1/1

== system mfordmodel_v1/iac_v04_001_001/activate_desired_rpm/hicam_rpm_request/fox_calcs/lookup_2d1 ==
  In1 : Inport
  Look-Up Table1 : Lookup  InputValues=calfunc.X  Table=calfunc.Y
  Saturation1 : Saturate  UpperLimit=max_x  LowerLimit=min_x
  Out1 : Outport
  wires:
  In1/1 -> Saturation1/1
  Saturation1/1 -> Look-Up Table1/1
  Look-Up Table1/1 -> Out1/1

== system mfordmodel_v1/iac_v04_001_001/activate_desired_rpm/hicam_rpm_request/fox_calcs/lookup_2d2 ==
  In1 : Inport
  Look-Up Table1 : Lookup  InputValues=calfunc.X  Table=calfunc.Y
  Saturation1 : Saturate  UpperLimit=max_x  LowerLimit=min_x
  Out1 : Outport
  wires:
  In1/1 -> Saturation1/1
  Saturation1/1 -> Look-Up Table1/1
  Look-Up Table1/1 -> Out1/1

== system mfordmodel_v1/iac_v04_001_001/activate_desired_rpm/hicam_rpm_request/fox_calcs/lookup_2d3 ==
  In1 : Inport
  Look-Up Table1 : Lookup  InputValues=calfunc.X  Table=calfunc.Y
  Saturation1 : Saturate  UpperLimit=max_x  LowerLimit=min_x
  Out1 : Outport
  wires:
  In1/1 -> Saturation1/1
  Saturation1/1 -> Look-Up Table1/1
  Look-Up Table1/1 -> Out1/1

== system mfordmodel_v1/iac_v04_001_001/activate_desired_rpm/hicam_rpm_request/fox_calcs/lookup_2d4 ==
  In1 : Inport
  Look-Up Table1 : Lookup  InputValues=calfunc.X  Table=calfunc.Y
  Saturation1 : Saturate  UpperLimit=max_x  LowerLimit=min_x
  Out1 : Outport
  wires:
  In1/1 -> Saturation1/1
  Saturation1/1 -> Look-Up Table1/1
  Look-Up Table1/1 -> Out1/1

== system mfordmodel_v1/iac_v04_001_001/activate_desired_rpm/hicam_rpm_request/fox_calcs/lookup_2d5 ==
  In1 : Inport
  Look-Up Table1 : Lookup  InputValues=calfunc.X  Table=calfunc.Y
  Saturation1 : Saturate  UpperLimit=max_x  LowerLimit=min_x
  Out1 : Outport
  wires:
  In1/1 -> Saturation1/1
  Saturation1/1 -> Look-Up Table1/1
  Look-Up Table1/1 -> Out1/1

== system mfordmodel_v1/iac_v04_001_001/activate_desired_rpm/hicam_rpm_request/hicam_calc/CONSTANT ==
  Constant : Constant  Value=const
  Out : Outport
  wires:
  Constant/1 -> Out/1
